simulink model "ConstantAngle"  (R2015a)
settings: Solver=ode45  StartTime=0.0  StopTime=10000  FixedStep=.1  RelTol=1e-10
values from neighbouring files (symbols this model uses):
  BurnStart = 1000    [Constants_simple.m]    (also in Solver_CA.m = (BurnStart_high+BurnStart_low)/2; Solver_GT.m = (BurnStart_high+BurnStart_low)/2)
  DryMass = 2236    [Constants_simple.m]
  FuelFlow = Thrust/(Isp*G0)    (= 17.7341950083)    [Constants_simple.m]
  g0 = 1.63    [Constants_simple.m]
  Starting_X_Speed = 100    [Constants_simple.m]
  Starting_Y_Speed = -25    [Constants_simple.m]
  StartingAlt = 1000    [Constants_simple.m]
  Theta_X = TWR'    [Solver_ThetaTable.m]    (also in Theta_Data.mat = [1.1 1.1898989899 1.2797979798 1.3696969697 1.4595959596 1.5)
  Theta_Y = (Vx./Vy)'    [Solver_ThetaTable.m]    (also in Theta_Data.mat = [0.0001 0.0103040711183 0.0207185139824 0.0313499020316 0.04)
  Theta_Z = Theta    [Solver_ThetaTable.m]    (also in Theta_Data.mat = [89.9994783103 89.9990867078 89.9987460673 89.9984537065 89.)
  Thrust = 60000    [Constants_simple.m]
  WetMass = 6235    [Constants_simple.m]
libraries: simulink x3
settings Model: Creator=raulm_000  LastModifiedBy=raulm_000

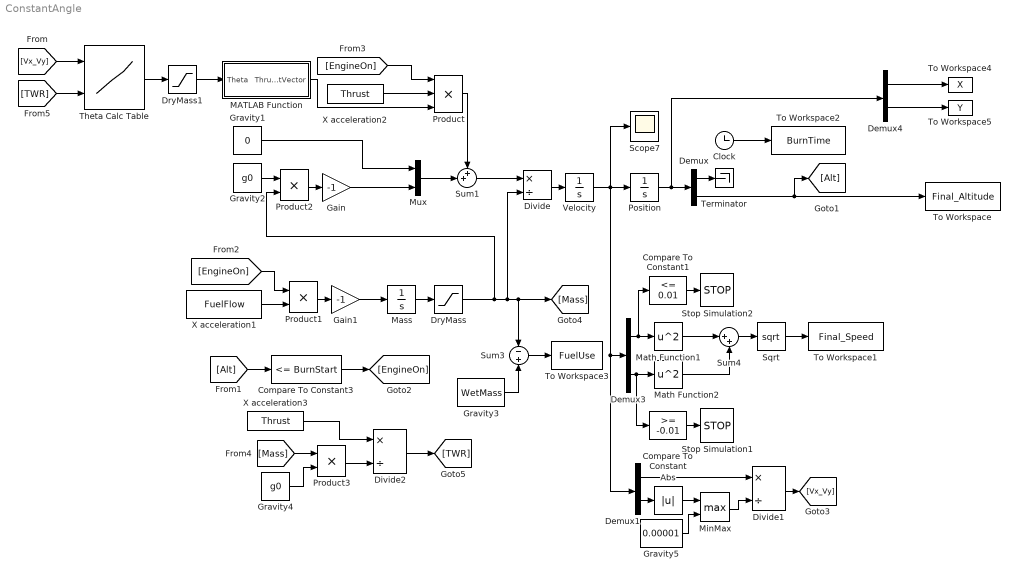
== system ConstantAngle ==
  Abs : Abs
  Clock : Clock
  Compare To Constant : simulink/Logic and Bit Operations/Compare To Constant  relop=>=  const=-0.01  OutDataTypeStr=boolean
  Compare To Constant1 : simulink/Logic and Bit Operations/Compare To Constant  relop=<=  const=0.01  OutDataTypeStr=boolean
  Compare To Constant3 : simulink/Logic and Bit Operations/Compare To Constant  relop=<=  const=BurnStart  OutDataTypeStr=boolean
  Demux{,1,3..4} (4 alike) : Demux  Outputs=2
  Divide : Product  Inputs=*/
  Divide1 : Product  Inputs=*/
  Divide2 : Product  Inputs=*/
  DryMass : Saturate  UpperLimit=inf  LowerLimit=DryMass
  DryMass1 : Saturate  UpperLimit=90  LowerLimit=0
  Gain : Gain  Gain=-1
  Gain1 : Gain  Gain=-1
  Gravity1 : Constant  Value=0
  Gravity2 : Constant  Value=g0
  Gravity3 : Constant  Value=WetMass
  Gravity4 : Constant  Value=g0
  Gravity5 : Constant  Value=0.00001
  MATLAB Function : MATLAB Function  TreatAsAtomicUnit=on
  Mass : Integrator  InitialCondition=WetMass
  Math Function1 : Math  Operator=square  SaturateOnIntegerOverflow=on
  Math Function2 : Math  Operator=square  SaturateOnIntegerOverflow=on
  MinMax : MinMax  Function=max  Inputs=2
  Mux : Mux  Inputs=2
  Position : Integrator  InitialCondition=[0,StartingAlt]
  Product : Product  Inputs=3
  Product1 : Product
  Product2 : Product
  Product3 : Product
  Scope7 : Scope
      settings: YMin=0.00075  YMax=0.00375  SaveName=ScopeData7
  Sqrt : Sqrt  SaturateOnIntegerOverflow=on
  Stop Simulation1 : Stop
  Stop Simulation2 : Stop
  Sum1 : Sum  Inputs=++|
  Sum3 : Sum  Inputs=-|+
  Sum4 : Sum  Inputs=|++
  Terminator : Terminator
  Theta Calc Table : Lookup_n-D  BreakpointsForDimension1=Theta_X  BreakpointsForDimension2=Theta_Y  BreakpointsForDimension3=[5, 7]  Table=Theta_Z  InternalRulePriority=Speed  RndMeth=Simplest  InputSameDT=on
  To Workspace : ToWorkspace  VariableName=Final_Altitude  SampleTime=-1
      settings: MaxDataPoints=1
  To Workspace1 : ToWorkspace  VariableName=Final_Speed  SampleTime=-1
      settings: MaxDataPoints=1
  To Workspace2 : ToWorkspace  VariableName=BurnTime  SampleTime=-1
      settings: MaxDataPoints=1
  To Workspace3 : ToWorkspace  VariableName=FuelUse  SampleTime=-1
      settings: MaxDataPoints=1
  To Workspace4 : ToWorkspace  VariableName=X  SampleTime=-1
  To Workspace5 : ToWorkspace  VariableName=Y  SampleTime=-1
  Velocity : Integrator  InitialCondition=[Starting_X_Speed,Starting_Y_Speed]
  X acceleration1 : Constant  Value=FuelFlow
  X acceleration2 : Constant  Value=Thrust
  X acceleration3 : Constant  Value=Thrust
  wires:
  Position/1 -> Demux4/1, Demux/1
  Gain/1 -> Mux/2
  Velocity/1 -> Scope7/1, Demux1/1, Demux3/1, Position/1
  Demux3/2 -> Compare To Constant/1, Math Function2/1
  Math Function1/1 -> Sum4/1
  Math Function2/1 -> Sum4/2
  Sum4/1 -> Sqrt/1
  Sqrt/1 -> To Workspace1/1
  Compare To Constant/1 -> Stop Simulation1/1
  X acceleration2/1 -> Product/2
  Demux3/1 -> Compare To Constant1/1, Math Function1/1
  Demux/1 -> Terminator/1
  Clock/1 -> To Workspace2/1
  Product/1 -> Sum1/1
  Compare To Constant1/1 -> Stop Simulation2/1
  Gain1/1 -> Mass/1
  Demux4/1 -> To Workspace4/1
  Demux4/2 -> To Workspace5/1
  Divide/1 -> Velocity/1
  Mass/1 -> DryMass/1
  DryMass/1 -> Product2/2, [Mass], Sum3/1, Divide/2
  Product1/1 -> Gain1/1
  X acceleration1/1 -> Product1/2
  Demux/2 -> [Alt], To Workspace/1
  [Alt] -> Compare To Constant3/1
  [EngineOn] -> Product1/1
  [EngineOn] -> Product/1
  Compare To Constant3/1 -> [EngineOn]
  Gravity2/1 -> Product2/1
  Product2/1 -> Gain/1
  Gravity1/1 -> Mux/1
  Mux/1 -> Sum1/2
  Sum1/1 -> Divide/1
  Sum3/1 -> To Workspace3/1
  Gravity3/1 -> Sum3/2
  Demux1/2 -> Abs/1
  Demux1/1 -> Divide1/1
  Divide1/1 -> [Vx_Vy]
  [Vx_Vy] -> Theta Calc Table/1
  [Mass] -> Product3/1
  Gravity4/1 -> Product3/2
  Product3/1 -> Divide2/2
  X acceleration3/1 -> Divide2/1
  Theta Calc Table/1 -> DryMass1/1
  DryMass1/1 -> MATLAB Function/1(Theta)
  MATLAB Function/1(ThrustVector) -> Product/3
  Abs/1 -> MinMax/1
  MinMax/1 -> Divide1/2
  Gravity5/1 -> MinMax/2
  Divide2/1 -> [TWR]
  [TWR] -> Theta Calc Table/2

== matlab function ConstantAngle/MATLAB Function ==
  data: Theta input; ThrustVector output
function ThrustVector = fcn(Theta)
%#codegen
X = -1*cosd(Theta);
Y = sind(Theta);
ThrustVector = [ X;Y ];
